simulink model "DuplicadorSIMU"  (R2024b)
settings: Solver=VariableStepAuto  StartTime=0.0  StopTime=0.01  RelTol=1e-3
settings Model: Creator=Aguirre  LastModifiedBy=Aguirre

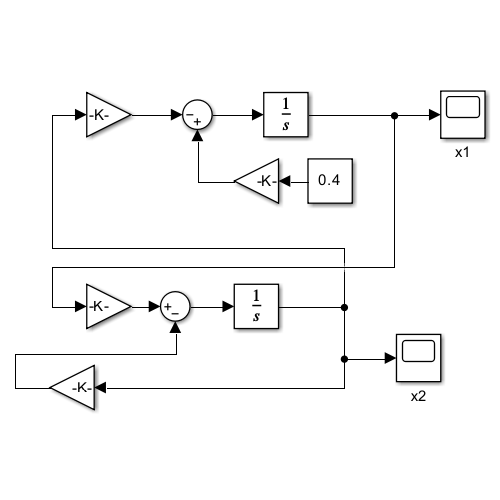
[thumbnail: Simulink's stored preview of the top-level diagram]
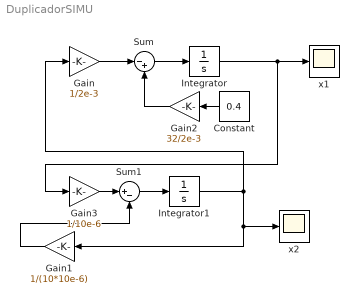
== system DuplicadorSIMU ==
  Constant : Constant  Value=0.4
  Gain : Gain  Gain=1/2e-3
  Gain1 : Gain  Gain=1/(10*10e-6)
  Gain2 : Gain  Gain=32/2e-3
  Gain3 : Gain  Gain=1/10e-6
  Integrator : Integrator
  Integrator1 : Integrator
  Sum : Sum  Inputs=|-+
  Sum1 : Sum  Inputs=|+-
  x1 : Scope
  x2 : Scope
  wires:
  Constant/1 -> Gain2/1
  Gain1/1 -> Sum1/2
  Integrator/1 -> x1/1, Gain3/1
  Sum/1 -> Integrator/1
  Gain/1 -> Sum/1
  Gain3/1 -> Sum1/1
  Sum1/1 -> Integrator1/1
  Gain2/1 -> Sum/2
  Integrator1/1 -> x2/1, Gain1/1, Gain/1
